simulink model "eml_asteroids"  (R2015a)
settings: Solver=FixedStepDiscrete  StartTime=0.0  StopTime=inf  FixedStep=1  RelTol=1e-3
StopFcn:
  | obj = findobj( 'Tag', 'asteroids_fig');
  | if ~isempty(obj),
  |    close(obj);
  | end;
libraries: simulink x2
(part 1 of 2)
CloseFcn:
  | rtwprivate ssgencode ModelCloseRequest asteroids_fixpt2
Description:
  | MATLAB fixed point version of the classic Asteroids game.
  | 
  | The classic Asteroids game. Even though it is purely fictitious (and not even physically
  | correct), it is nevertheless a complicated dynamic system including collisions,
  | rotating polygons and gaming logic.
  | 
  | This version is using MATLAB Function block and fixed point to demonstrate that all the
  | computations can be done without use of floating point math. Only the "Plot" block
  | in this model contains doubles for displaying and figure handling.
  | 
  | The orange blocks are the core of the simulation and the yellow block is responsible for
  | displaying the results. The blue blocks are managing the input controls, i.e. the space
  | ship rotation, thrust and firing.
  | 
  | Except for the "Plot" visualization block's use of plotting routines, all of the
  | MATLAB Function blocks in this model support code generation with
  | Real-Time Workshop and Real-Time Workshop Embedded Coder.
  | 
  |   Demo Requirements
  | 
  | During this demonstration, Simulink generates code for the simulation in a Simulink
  | project directory created in the current working directory (pwd). If you do not want
  | to affect the current directory (or if you cannot) generate files in this directory, you
  | should change your working directory.
settings Model: CovSFcnEnable=off  ExtModeAutoUpdateStatusClock=off  Creator=The MathWorks, Inc.  LastModifiedBy=ktrinh
settings DataIOCC: SaveFormat=Structure
settings OptimizationCC: ExpressionDepthLimit=2147483647  InitFltsAndDblsToZero=on  EfficientMapNaN2IntZero=off  BufferReusableBoundary=off
settings DebuggingCC: SaveWithParameterizedLinksMsg=none  UnderspecifiedInitializationDetection=Classic  MergeDetectMultiDrivingBlocksExec=none  CheckExecutionContextPreStartOutputMsg=on  CheckExecutionContextRuntimeOutputMsg=on  SignalResolutionControl=TryResolveAllWithWarning  SolverPrmCheckMsg=warning  MultiTaskDSMMsg=warning  MultiTaskCondExecSysMsg=none  SigSpecEnsureSampleTimeMsg=none  IntegerOverflowMsg=none  FcnCallInpInsideContextMsg=EnableAllAsWarning  BusObjectLabelMismatch=none  StateNameClashWarn=warning  IntegerSaturationMsg=none
settings SFSimCC: SimParseCustomCode=off
settings GRTTargetCC: TargetFcnLib=ansi_tfl_tmw.mat  CombineOutputUpdateFcns=off  GRTInterface=on

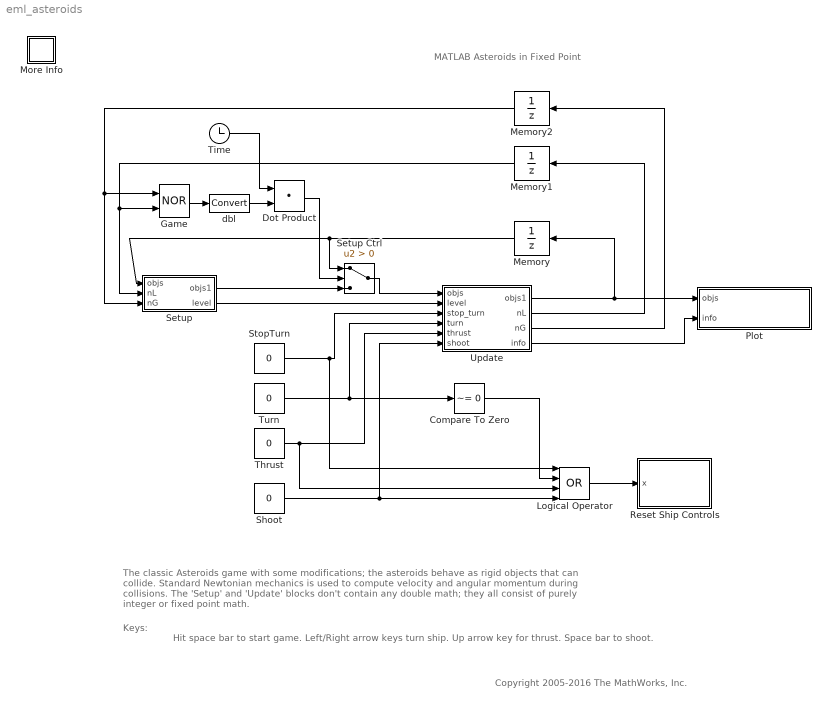
== system eml_asteroids ==
  note: MATLAB Asteroids in Fixed Point
  note: The classic Asteroids game with some modifications; the asteroids behave as rigid objects that can collide.
      | Standard Newtonian mechanics is used to compute velocity and angular momentum during collisions. The 'Setup'
      | and 'Update' blocks don't contain any double math; they all consist of purely integer or fixed point math.
  note: Hit space bar to start game. Left/Right arrow keys turn ship. Up arrow key for thrust.
      | Space bar to shoot.
  note: Keys:
  note: Copyright 2005-2016 The MathWorks, Inc.
  Compare To Zero : simulink/Logic and Bit Operations/Compare To Zero  relop=~=  OutDataTypeStr=boolean  ZeroCross=off
  Dot Product : DotProduct  InputSameDT=on  OutDataTypeStr=Inherit: Inherit via internal rule
  Game : Logic  Operator=NOR  AllPortsSameDT=off  OutDataTypeStr=boolean
  Logical Operator : Logic  Operator=OR  Inputs=4  AllPortsSameDT=off  OutDataTypeStr=boolean
  Memory : UnitDelay  SampleTime=-1
  Memory1 : UnitDelay  SampleTime=-1
  Memory2 : UnitDelay  SampleTime=-1
  More Info : Subsystem
      mask Display: disp('?')
  Plot : MATLAB Function  TreatAsAtomicUnit=on
      settings: PermitHierarchicalResolution=ParametersOnly
  Reset Ship Controls : MATLAB Function  TreatAsAtomicUnit=on
      settings: PermitHierarchicalResolution=ParametersOnly
  Setup : Subsystem
  Setup Ctrl : Switch  Criteria=u2 > Threshold  ZeroCross=off
  Shoot : Constant  Value=0  OutDataTypeStr=boolean
  StopTurn : Constant  Value=0  OutDataTypeStr=boolean
  Thrust : Constant  Value=0  OutDataTypeStr=boolean
  Time : Clock
  Turn : Constant  Value=0  OutDataTypeStr=int32
  Update : Subsystem
  dbl : DataTypeConversion
  wires:
  Time/1 -> Dot Product/1
  Memory/1 -> Setup Ctrl/1, Setup/1(objs)
  Setup Ctrl/1 -> Update/1(objs)
  Turn/1 -> Compare To Zero/1, Update/4(turn)
  Thrust/1 -> Logical Operator/3, Update/5(thrust)
  Logical Operator/1 -> Reset Ship Controls/1(x)
  StopTurn/1 -> Logical Operator/1, Update/3(stop_turn)
  Shoot/1 -> Logical Operator/4, Update/6(shoot)
  Update/1(objs1) -> Plot/1(objs), Memory/1
  Update/2(nL) -> Memory1/1
  Memory1/1 -> Game/2, Setup/2(nL)
  Dot Product/1 -> Setup Ctrl/2
  dbl/1 -> Dot Product/2
  Game/1 -> dbl/1
  Compare To Zero/1 -> Logical Operator/2
  Setup/1(objs1) -> Setup Ctrl/3
  Memory2/1 -> Game/1, Setup/3(nG)
  Update/3(nG) -> Memory2/1
  Update/4(info) -> Plot/2(info)
  Setup/2(level) -> Update/2(level)

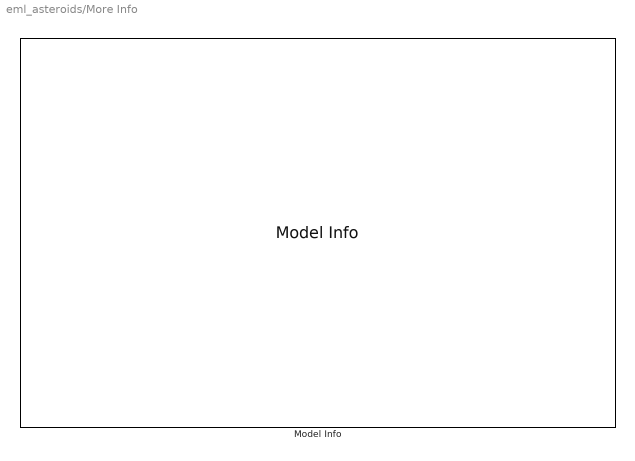
== system eml_asteroids/More Info ==
  Model Info : simulink/Model-Wide Utilities/Model Info  Frame=on  DisplayStringWithTags=|  HorizontalTextAlignment=Left  LeftAlignmentValue=0.02
      | Model Description:
      | -------------------
      | 
      | %<Description>

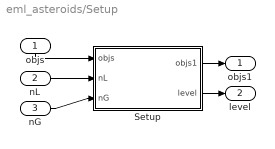
== system eml_asteroids/Setup ==
  objs : Inport
  nL : Inport  Port=2
  nG : Inport  Port=3
  Setup : MATLAB Function  TreatAsAtomicUnit=on
      settings: PermitHierarchicalResolution=ParametersOnly
  objs1 : Outport
  level : Outport  Port=2
  wires:
  objs/1 -> Setup/1(objs)
  nL/1 -> Setup/2(nL)
  nG/1 -> Setup/3(nG)
  Setup/1(objs1) -> objs1/1
  Setup/2(level) -> level/1

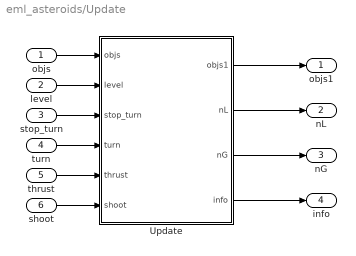
== system eml_asteroids/Update ==
  objs : Inport
  level : Inport  Port=2
  stop_turn : Inport  Port=3
  turn : Inport  Port=4
  thrust : Inport  Port=5
  shoot : Inport  Port=6
  Update : MATLAB Function  TreatAsAtomicUnit=on
      settings: PermitHierarchicalResolution=ParametersOnly
  objs1 : Outport
  nL : Outport  Port=2
  nG : Outport  Port=3
  info : Outport  Port=4
  wires:
  stop_turn/1 -> Update/3(stop_turn)
  turn/1 -> Update/4(turn)
  thrust/1 -> Update/5(thrust)
  shoot/1 -> Update/6(shoot)
  objs/1 -> Update/1(objs)
  Update/1(objs1) -> objs1/1
  level/1 -> Update/2(level)
  Update/2(nL) -> nL/1
  Update/3(nG) -> nG/1
  Update/4(info) -> info/1

== matlab function eml_asteroids/Setup/Setup ==
  data: objs input fixdt('sfix32_En12'); nL input boolean; objs1 output fixdt('sfix32_En12'); nG input boolean; level output fixdt('sfix32_En12')
function [objs1,level] = setup(objs,nL,nG)

% nL = nextLevel

my_fimath = fimath('MaxProductWordLength',32,'MaxSumWordLength',32,...
                   'ProductFractionLength',12,'ProductMode','SpecifyPrecision',...
                   'SumFractionLength',12,'SumMode','SpecifyPrecision');
my_fitype = numerictype(1,32,12);

persistent level0;
persistent objs0;

maxobjs = 64;

initial = false;

if isempty(level0)
    level0 = fi(0,my_fitype,my_fimath);
    nL = true;
    initial = true;
end

if nG
    level0 = fi(0,my_fitype,my_fimath);
    nL = true;
end

if nL
    level0 = level0 + 1;
end

level = level0;

objs0 = fi(objs,my_fitype,my_fimath);

if isempty(objs0)
    objs0 = fi(zeros(11,maxobjs),my_fitype,my_fimath);
end

if nG
    % Delete all objects that is not a ship
    for i = 1:maxobjs
        if objs0(1,i) ~= 2 % ship id
            objs0(1,i) = 0;
        end
    end
end

if nL
    if level0 < 5
        level0_int = fi(level0,numerictype(1,16,0));
        n = int32(level0_int) + 1;
    else
        n = int32(5);
    end
 
    if initial
        n = int32(20);
    end
 
    for z = int32(1):n
        objs0 = add_asteroid(objs0,initial);
    end
       
    % Move objects so two objects never collide
    
     for z = int32(1):n
         x = objs0(2,z);
         y = objs0(3,z);
         r = objs0(10,z);
         q = true;
         while q
             c = false;
             for k = int32(1):n
                 if z ~= k
                     xk = objs0(2,k);
                     yk = objs0(3,k);
                     rk = objs0(10,k);
                     dx = x-xk;
                     ddx = x*xk;
                     dy = y-yk;
                     rrk = r+rk;
                     if dx*dx+dy*dy < rrk*rrk
                         c = true;
                         break;
                     end
                 end
             end
             q = c;
             if q
                 x = fi(400 * fi_rand(),my_fitype,my_fimath);
                 y = fi(400 * fi_rand(),my_fitype,my_fimath);
                 objs0(2,z) = x;
                 objs0(3,z) = y;
             end
         end
     end  
end
objs1 = objs0;

function [objs1,index] = add_object(objs,id,r)
    my_fimath = fimath('MaxProductWordLength',32,'MaxSumWordLength',32);
    my_fitype = numerictype(1,32,20);

    x = 400 * fi_rand();
    y = 400 * fi_rand();
    arg = fi_rand()*2*pi;
    vx = fi_rand()*6 - 3;
    vy = fi_rand()*6 - 3;
    varg = fi_rand()*0.2 - 0.1;
    collidable = 1;
    i = add_new(objs);
    col = double('w');
    cnt = 0;
    objs(:,i) = fi([id x y arg vx vy varg collidable col r cnt]',my_fitype,my_fimath);
    objs1 = objs;
    index = i;

function objs1 = add_asteroid(objs,initial)
    r = fi_rand() * 15 + 8;
    if ~initial
        r(:) = 30;
    end 
    [objs1,i] = add_object(objs,int32(1),r);
    objs1(5,i) = objs1(5,i)*0.1;
    objs1(6,i) = objs1(6,i)*0.1;
    objs1(7,i) = objs1(7,i)*0.1;

function r = fi_rand()

persistent state;

my_fimath0 = fimath('MaxProductWordLength',32,'MaxSumWordLength',32,...
                    'ProductFractionLength',32,'ProductMode','SpecifyPrecision',...
                    'SumFractionLength',32,'SumMode','SpecifyPrecision',...
                    'OverflowMode','wrap');
my_fitype0 = numerictype(0,32,32);
                
my_fimath = fimath('MaxProductWordLength',32,'MaxSumWordLength',32,...
                   'ProductFractionLength',12,'ProductMode','SpecifyPrecision',...
                   'SumFractionLength',12,'SumMode','SpecifyPrecision');

my_fitype = numerictype(1,32,12);

if isempty(state)
    state = fi(0,my_fitype0,my_fimath0);
end

state = state * 34567.27491803 + 43178.421727917;

r = fi(state,my_fitype,my_fimath);

function index = add_new(objs)
    maxobjs = 64;
    index = int32(-1);
    for i = 1:maxobjs,
        if objs(1,i) == 0,
            index = int32(i);
            return
        end
    end

== matlab function eml_asteroids/Update/Update ==
  settings: updateMethod=DISCRETE
  data: objs input fixdt('sfix32_En12') size=[11,64]; level input fixdt('sfix32_En12'); stop_turn input boolean; turn input int32 size=1; objs1 output fixdt('sfix32_En12') size=[11,64]; nL output boolean; nG output boolean; info output fixdt('sfix32_En12'); thrust input boolean; shoot input boolean
function [objs1,nL,nG,info] = update(objs, level, stop_turn, turn, thrust, shoot)

persistent stop;
persistent thrust_cnt;
persistent turn_cnt;
persistent turn_dir;
persistent ship_cnt;
persistent ship_destroyed_cnt;
persistent level_complete_cnt;
persistent score;

my_fimath = fimath('MaxProductWordLength',32,'MaxSumWordLength',32,...
                   'ProductFractionLength',12,'ProductMode','SpecifyPrecision',...
                   'SumFractionLength',12,'SumMode','SpecifyPrecision');
my_fitype = numerictype(1,32,12);

objs1 = fi(objs,my_fitype,my_fimath);
nL = false;
nG = false;

if isempty(score)
    score = fi(0,my_fitype,my_fimath);
end

%
% stop is used for debugging. It is convenient to "freeze" the
% updates.
%
if isempty(stop)
    stop = false;
end

if isempty(ship_cnt)
    ship_cnt = fi(0,my_fitype,my_fimath);
end

if isempty(thrust_cnt)
    thrust_cnt = fi(0,my_fitype,my_fimath);
end

if isempty(turn_cnt) || stop_turn
    turn_cnt = fi(0,my_fitype,my_fimath);
    turn_dir = int32(0);
end

if isempty(ship_destroyed_cnt)
    ship_destroyed_cnt = fi(0,my_fitype,my_fimath);
end

if isempty(level_complete_cnt)
    level_complete_cnt = fi(0,my_fitype,my_fimath);
end

if level_complete_cnt > 200
    level_complete_cnt = fi(0,my_fitype,my_fimath);
    nL = true;
end

if turn ~= 0
    turn_cnt = fi(3,my_fitype,my_fimath);
    turn_dir = turn;
end

info = [level ship_cnt score];

if stop
    return
end

min_x = fi(0,my_fitype,my_fimath) - 20;
max_x = fi(400,my_fitype,my_fimath) + 20;
min_y = fi(0,my_fitype,my_fimath) - 20;
max_y = fi(400,my_fitype,my_fimath) + 20;
width = max_x - min_x;
height = max_y - min_y;

origin_x = (max_x + min_x) * 0.5;
origin_y = (max_y + min_y) * 0.5;

if ship_destroyed_cnt > 0
    ship_destroyed_cnt = ship_destroyed_cnt - 1;
end

% Make sure thrust is at the same position as ship
maxobjs = int32(64);

ship_index = int32(0);
thrust_index = int32(0);
no_asteroids = true;
for i = int32(1):maxobjs
    if objs1(1,i) == 2 % space ship id
        ship_index = int32(i);
    end
    if objs1(1,i) == 5 % thrust id
        thrust_index = int32(i);
    end
    if objs1(1,i) == 1 % asteroid id
        no_asteroids = false;
    end
end

ship_exists = ship_index > 0;

if ship_destroyed_cnt <= 0 && ship_cnt > 0 && ~ship_exists
    if is_space_empty(objs1,origin_x,origin_y,40)
        [objs1,ship_index] = add_ship(objs1,origin_x,origin_y);
        ship_cnt = ship_cnt - 1;
        ship_exists = true;
    end
end

if ~ship_exists && shoot && ship_cnt == 0
    ship_cnt = fi(3,my_fitype,my_fimath);
    score = fi(0,my_fitype,my_fimath);
    nG = true;
end

if thrust ~= 0 && thrust_cnt == 0 && ship_index > 0
    thrust_cnt = fi(7,my_fitype,my_fimath);
    [objs1,thrust_index] = add_thrust(objs1);
end

if no_asteroids && ship_index > 0
    level_complete_cnt = level_complete_cnt + 1;
end
    
if thrust_index > 0 && ship_index > 0
    objs1(2:7,thrust_index) = objs1(2:7,ship_index);
end

% fprintf(1,'i=%d id=%d r=%d\n', i, double(objs1(1,i)), double(objs1(2,i)));

%
% Start updating all objects
%

for i = int32(1):maxobjs
    id = objs1(1,i);
%    fprintf(1,'i=%d id=%d r=%d\n', i, double(id), double(objs1(1,i)));
    if id == 0 % marked deleted
        continue
    end
    x = objs1(2,i);
    y = objs1(3,i);
    arg = objs1(4,i);
    vx = objs1(5,i);
    vy = objs1(6,i);
    varg = objs1(7,i);
    collidable = objs1(8,i);
    color = objs1(9,i);
    r = objs1(10,i);
    cnt = objs1(11,i);
        
    if cnt > 0
        cnt = cnt - 1;
        objs1(11,i) = cnt;
        if cnt <= 0 % delete object
            objs1(1,i) = 0;
            continue
        end
    end
    
    if id == 2 % space ship
        
        if turn_cnt > 0
            turn_cnt = turn_cnt - 1;
            if turn_dir == -1
                varg = fi(-0.1,numerictype(varg),fimath(varg));
            elseif turn_dir == 1
                varg = fi(0.1,numerictype(varg),fimath(varg));
            else
                varg = fi(0,numerictype(varg),fimath(varg));
            end
        else
            varg = fi(0,numerictype(varg),fimath(varg));
        end
        objs1(7,i) = varg;
        
        if thrust_cnt > 0
            thrust_cnt = thrust_cnt - 1;            
            if thrust_cnt == 6
                vx = vx + cos(arg)*0.3;
                vy = vy + sin(arg)*0.3;
            end
            objs1(5,i) = vx;
            objs1(6,i) = vy;
        end
        
        if shoot ~= 0 && ship_exists
            missile_cnt = fi(0,my_fitype,my_fimath);
            for j = int32(1):maxobjs
                if objs(1,j) == 3
                    missile_cnt = missile_cnt + 1;
                end
            end
            if missile_cnt < 3
                mx = x + (r+2)*cos(arg);
                my = y + (r+2)*sin(arg);
                mvx = vx + 3*cos(arg);
                mvy = vy + 3*sin(arg);
                objs1 = add_missile(objs1,mx,my,mvx,mvy,arg);
                missile_cnt = missile_cnt + 1;
            end
        end
    end
    
    arg = arg + varg;
    x = x + vx;
    y = y + vy;    
    
    while arg >= 2*pi, arg = arg - 2*pi; end
    while arg < 0, arg = arg + 2*pi; end

    objs1(2,i) = x;
    objs1(3,i) = y;
    objs1(4,i) = arg;
    
    while x > max_x
        x = x - width;
        objs1(2,i) = x;
        objs1 = move_to_empty_space(objs1,i,int32(0),int32(10),min_x,max_x,min_y,max_y);
    end
    while x < min_x
        x = x + width;
        objs1(2,i) = x;
        objs1 = move_to_empty_space(objs1,i,int32(0),int32(10),min_x,max_x,min_y,max_y);
    end
    while y > max_y
        y = y - height; 
        objs1(3,i) = y;
        objs1 = move_to_empty_space(objs1,i,int32(10),int32(0),min_x,max_x,min_y,max_y);
    end
    while y < min_y
        y = y + height; 
        objs1(3,i) = y;
        objs1 = move_to_empty_space(objs1,i,int32(10),int32(0),min_x,max_x,min_y,max_y);
    end
    
    [xs ys n] = get_object_data(objs1(:,i));
    
    for j = int32(1):maxobjs
        if objs1(1,j) == 0 % object marked deleted
            continue
        end
        collidable_j = objs1(8,j);
        if i ~= j && collidable ~= 0 && collidable_j ~= 0 && collides(objs1(:,i),objs1(:,j))

            if (objs1(1,i) == 3 && objs1(1,j) == 1) || ...
               (objs1(1,i) == 1 && objs1(1,j) == 3) % if missile + asteroid
                [dir_x,dir_y] = get_any_dir;
                if objs1(1,i) == 3
                    x0 = objs1(2,i); y0 = objs1(3,i);
                    objs1(:,i) = objs1(:,j);
                else
                    x0 = objs1(2,j); y0 = objs1(3,j);
                    objs1(:,j) = objs1(:,i);
                end
                vel = fi(2,my_fitype,my_fimath);
                vel = vel*fi_rand() + 1;
                asteroid_size = objs1(10,i);
                objs1(10,i) = objs1(10,i) * 0.5;
                objs1(10,j) = objs1(10,i);
                if objs1(10,i) < 4
                    objs1(1,i) = 0;
                    objs1(1,j) = 0;
                else
                    objs1(4,i) = objs1(4,i) + vel*dir_x;
                    objs1(5,i) = objs1(5,i) + vel*dir_y;
                    objs1(4,j) = objs1(4,j) - vel*dir_x;
                    objs1(5,j) = objs1(5,j) - vel*dir_y;
                    objs1(2,i) = objs1(2,i) + objs1(10,i)*dir_x;
                    objs1(3,i) = objs1(3,i) + objs1(10,i)*dir_y;
                    objs1(2,j) = objs1(2,j) - objs1(10,i)*dir_x;
                    objs1(3,j) = objs1(3,j) - objs1(10,i)*dir_y;
                end
                objs1 = add_explosion(objs1,x0,y0,int32(40));

                if asteroid_size >= 25
                    score = score + 20;
                elseif asteroid_size >= 13
                    score = score + 50;
                else
                    score = score + 100;
                end

                continue
            end

            ship_index = int32(-1);
            ship_vx = fi(0,my_fitype,my_fimath);
            ship_vy = fi(0,my_fitype,my_fimath);
            ship_varg = fi(0,my_fitype,my_fimath);
            if (objs1(1,i) == 2 || objs1(1,j) == 2) % if ship + something else
                if objs1(1,i) == 2
                    ship_index = int32(i);
                else
                    ship_index = int32(j);
                end
                ship_vx = objs1(5,ship_index);
                ship_vy = objs1(6,ship_index);
                ship_varg = objs1(7,ship_index);
            end

%            objs1(9,i) = double('r');
            [objs1(:,i),objs1(:,j)] = do_collision(objs1(:,i),objs1(:,j));

            if ship_index ~= -1
                ship_vx = ship_vx - objs1(5,ship_index);
                ship_vy = ship_vy - objs1(6,ship_index);
                ship_varg = ship_varg - objs1(7,ship_index);
                ship_vr = ship_varg*ship_r();
                % If ship gained to much energy in the collison we'll destroy it
                delta = sqrt(ship_vx*ship_vx+ship_vy*ship_vy+ship_varg*ship_varg);
                if delta >= 0.2 % Empirically tested (it feels right)
                    objs1(1,ship_index) = 0; % remove ship
                    ship_destroyed_cnt = fi(100,my_fitype,my_fimath);
                    objs1 = add_explosion(objs1,objs1(2,ship_index),objs1(3,ship_index),int32(100));
                end
            end
            
%            stop = true;
            break
        else
%            objs1(9,i) = double('w');
        end
    end
end

function b = is_space_empty(objs,x,y,r)
    maxobjs = 64;
    for j = 1:maxobjs
        if objs(8,j) ~= 0 && objs(1,j) ~= 0 ...
            radius = objs(10,j);
            dx = objs(2,j) - x;
            dy = objs(3,j) - y;
            if dx*dx+dy*dy < (r+radius)*(r+radius)
                b = false;
                return
            end
        end
    end
    b = true;

function objs1 = move_to_empty_space(objs,obj_i,dx,dy,min_x,max_x,min_y,max_y)
    maxobjs = 64;
    width = max_x - min_x;
    height = max_y - min_y;
    objs1 = objs;
    some_collision = true;
    wraps = int32(0);
    if objs1(8,obj_i) == 0
        return
    end
    while some_collision && wraps < 2
        some_collision = false;
        for j = 1:maxobjs
            if objs1(1,j) == 0
                continue
            end
            if obj_i ~= j && objs1(8,j) ~= 0 && collides(objs1(:,obj_i),objs1(:,j))
                x = objs1(2,obj_i);
                y = objs1(3,obj_i);
                x = x + dx;
                y = y + dy;
                while x > max_x, x = x - width; wraps = wraps + 1; end
                while x < min_x, x = x + width; wraps = wraps + 1; end
                while y > max_y, y = y - height; wraps = wraps + 1; end
                while y < min_y, y = y + height; wraps = wraps + 1; end
                objs1(2,obj_i) = x;
                objs1(3,obj_i) = y;
                some_collision = true;
            end
        end
    end

function r = fi_rand()

persistent state;

my_fimath0 = fimath('MaxProductWordLength',32,'MaxSumWordLength',32,...
                    'ProductFractionLength',32,'ProductMode','SpecifyPrecision',...
                    'SumFractionLength',32,'SumMode','SpecifyPrecision',...
                    'OverflowMode','wrap');
my_fitype0 = numerictype(0,32,32);
                
my_fimath = fimath('MaxProductWordLength',32,'MaxSumWordLength',32,...
                   'ProductFractionLength',12,'ProductMode','SpecifyPrecision',...
                   'SumFractionLength',12,'SumMode','SpecifyPrecision');

my_fitype = numerictype(1,32,12);

if isempty(state)
    state = fi(0,my_fitype0,my_fimath0);
end

state = state * 34567.27491803 + 43178.421727917;

r = fi(state,my_fitype,my_fimath);

%
% get any direction
%


function [dx,dy] = get_any_dir
    arg = fi_rand()*2*pi;
    dx = cos(arg);
    dy = sin(arg);

%
% do_collision
%
% Compute new momentum for objects
%

function [obj1,obj2] = do_collision(obj1,obj2)

[px,py] = collision_point(obj1,obj2);
[nx,ny] = collision_normal(obj1,obj2);
n = [nx ny];
p = [px py];

c = true;

cnt = int32(0);

while c
    [obj1,obj2] = do_collision0(obj1,obj2,p,n);

    c = collides(obj1,obj2);
    if c
        q = fi_rand();
        arg = fi(q,numerictype(p),fimath(p)) * 2 * pi;
        n = n * [cos(arg) sin(arg); -sin(arg) cos(arg)];
        cnt = cnt + 1;
        if cnt > 10
%            disp('failed!');
            break;
        end
    end
end

function [obj1,obj2] = do_collision0(obj1,obj2,p,n)

px = p(1);
py = p(2);
nx = n(1);
ny = n(2);

i1 = get_inertia(obj1);
m1 = get_mass(obj1);
x1 = obj1(2);
y1 = obj1(3);
vx1 = obj1(5);
vy1 = obj1(6);
w1 = obj1(7);
r1 = obj1(10);

i2 = get_inertia(obj2);
m2 = get_mass(obj2);
x2 = obj2(2);
y2 = obj2(3);
vx2 = obj2(5);
vy2 = obj2(6);
w2 = obj2(7);
r2 = obj2(10);

%
% Before we do anything, let's undo the collision point so
% objects don't get stuck because we compute the collision
% normal slightly wrong.
%

obj1(2) = obj1(2) - vx1;
obj1(3) = obj1(3) - vy1;
obj1(4) = obj1(4) - w1;
obj2(2) = obj2(2) - vx2;
obj2(3) = obj2(3) - vy2;
obj2(4) = obj2(4) - w2;


v1 = [vx1 vy1];
v2 = [vx2 vy2];
r1p = [px-x1 py-y1];
r2p = [px-x2 py-y2];

w1r1p = cross([0 0 w1],[r1p 0]);
w2r2p = cross([0 0 w2],[r2p 0]);

v1p = v1 + w1r1p(1:2);
v2p = v2 + w2r2p(1:2);

v21 = v1p - v2p;

e = 1.00;

xx1 = cross([r1p 0],[n 0]);
xx2 = cross([r2p 0],[n 0]);

j1 = (-(1+e)*v21) * n';
j2 = divide(numerictype(m1),1,m1) + ...
     divide(numerictype(m2),1,m2) + ...
     divide(numerictype(xx1),(xx1 * xx1'),i1) + ...
     divide(numerictype(xx2),(xx2 * xx2'),i2);

j = divide(numerictype(j1),j1,j2);

new_v1 = v1 + j * divide(numerictype(n),n,m1);
new_v2 = v2 - j * divide(numerictype(n),n,m2);

new_w1 = w1 + divide(numerictype(j),j,i1)*xx1(3);
new_w2 = w2 - divide(numerictype(j),j,i2)*xx2(3);

obj1(5) = new_v1(1);
obj1(6) = new_v1(2);
obj1(7) = new_w1;

obj2(5) = new_v2(1);
obj2(6) = new_v2(2);
obj2(7) = new_w2;

obj1(2) = obj1(2) + new_v1(1);
obj1(3) = obj1(3) + new_v1(2);
obj1(4) = obj1(4) + new_w1;

obj2(2) = obj2(2) + new_v2(1);
obj2(3) = obj2(3) + new_v2(2);
obj2(4) = obj2(4) + new_w2;
   
%
% add object
%

function [objs1,index] = add_object(objs,id,r,x,y,vx,vy,arg,col)
    my_fimath = fimath('MaxProductWordLength',32,'MaxSumWordLength',32,...
                       'ProductFractionLength',12,'ProductMode','SpecifyPrecision',...
                       'SumFractionLength',12,'SumMode','SpecifyPrecision');
    my_fitype = numerictype(1,32,12);
    varg = 0;
    collidable = 1;
    index = add_new(objs);
    if nargin < 9
        ficol = fi(int32('w'),my_fitype,my_fimath);
    else
        ficol = fi(int32(col),my_fitype,my_fimath);
    end
    objs(:,index) = fi([id x y arg vx vy varg collidable ficol r -1]',my_fitype,my_fimath);
    objs1 = objs;

function [objs1,index] = add_ship(objs,x,y)
    my_fimath = fimath('MaxProductWordLength',32,'MaxSumWordLength',32,...
                       'ProductFractionLength',12,'ProductMode','SpecifyPrecision',...
                       'SumFractionLength',12,'SumMode','SpecifyPrecision');
    my_fitype = numerictype(1,32,12);
    [objs1,index] = add_object(objs,2,15,x,y,0,0,fi(pi/2,my_fitype,my_fimath),'g');

function [objs1,index] = add_thrust(objs)
    [objs1,index] = add_object(objs,5,15,0,0,0,0,0,'y');
    objs1(11,index) = 15; % Life time
    objs1(8,index) = 0; % not collidable
    
function objs1 = add_missile(objs,x,y,vx,vy,arg)
    [objs1,index] = add_object(objs,3,4,x,y,vx,vy,arg,'y');
    objs1(11,index) = 50; % Life time

function obj = new_explosion(x,y,n)
    my_fimath = fimath('MaxProductWordLength',32,'MaxSumWordLength',32,...
                       'ProductFractionLength',12,'ProductMode','SpecifyPrecision',...
                       'SumFractionLength',12,'SumMode','SpecifyPrecision');
    my_fitype = numerictype(1,32,12);
    obj = fi([4 x y 0 0 0 0 0 double('w') n 2]',my_fitype,my_fimath);
    
function objs1 = add_explosion(objs,x,y,n)
    index = add_new(objs);
    obj = new_explosion(x,y,n);
    objs1 = objs;
    objs1(:,index) = obj;
    
function index = add_new(objs)
    my_fimath = fimath('MaxProductWordLength',32,'MaxSumWordLength',32,...
                       'ProductFractionLength',12,'ProductMode','SpecifyPrecision',...
                       'SumFractionLength',12,'SumMode','SpecifyPrecision');
    my_fitype = numerictype(1,32,12);
    maxobjs = 64;
    index = int32(-1);
    for i = 1:maxobjs,
        if objs(1,i) == 0
            index = int32(i);
            return
        end
    end
    feval('error','overflow objects');

function n = get_number(objs)    
    n = add_new(objs);

%
% get_object_data
%
% Get point data given object
%
function [xs ys n] = get_object_data(obj)

id = obj(1);
x = obj(2);
y = obj(3);
arg = obj(4);
r = obj(10);

xs = fi([0 0 0 0 0 0 0 0 0 0 0 0 0 0 0 0],numerictype(x),fimath(x));
ys = fi([0 0 0 0 0 0 0 0 0 0 0 0 0 0 0 0],numerictype(y),fimath(y));
n = int32(0);
if id == 1,
    asteroid_x0 = asteroid_x();
    asteroid_y0 = asteroid_y();
    asteroid_r0 = asteroid_r();
    f = divide(numerictype(r),r,asteroid_r0);
    n = int32(size(asteroid_x0,1));
    xs(1:n) = x + f * asteroid_x0 * cos(arg) - f * asteroid_y0 * sin(arg);
    ys(1:n) = y + f * asteroid_x0 * sin(arg) + f * asteroid_y0 * cos(arg);
elseif id == 2
    ship_x0 = ship_x();
    ship_y0 = ship_y();
    ship_r0 = ship_r();
    f = divide(numerictype(r),r,ship_r0);
    n = int32(size(ship_x0,1));
    xs(1:n) = x + f * ship_x0 * cos(arg) - f * ship_y0 * sin(arg);
    ys(1:n) = y + f * ship_x0 * sin(arg) + f * ship_y0 * cos(arg);    
else % id == 3
    missile_x0 = missile_x();
    missile_y0 = missile_y();
    missile_r0 = missile_r();
    f = divide(numerictype(r),r,missile_r0);
    n = int32(size(missile_x0,1));
    xs(1:n) = x + f * missile_x0 * cos(arg) - f * missile_y0 * sin(arg);
    ys(1:n) = y + f * missile_x0 * sin(arg) + f * missile_y0 * cos(arg);    
end

%
% asteroid_x
% asteroid_y
%
% Returning asteroid x and y data
%

function r = asteroid_x
    my_fimath = fimath('MaxProductWordLength',32,'MaxSumWordLength',32,...
                       'ProductFractionLength',12,'ProductMode','SpecifyPrecision',...
                       'SumFractionLength',12,'SumMode','SpecifyPrecision');
    my_fitype = numerictype(1,32,12);
    r = fi([2 10 20 17 7 16 12 -7 -17 -21 -14 -8 -7]',my_fitype,my_fimath);

function r = asteroid_y
    my_fimath = fimath('MaxProductWordLength',32,'MaxSumWordLength',32,...
                       'ProductFractionLength',12,'ProductMode','SpecifyPrecision',...
                       'SumFractionLength',12,'SumMode','SpecifyPrecision');
    my_fitype = numerictype(1,32,12);
    r = fi([18 22 5 -4 -6 -10 -17 -19 -13 3 17 11 23]',my_fitype,my_fimath);

function r = asteroid_r
    my_fimath = fimath('MaxProductWordLength',32,'MaxSumWordLength',32,...
                       'ProductFractionLength',12,'ProductMode','SpecifyPrecision',...
                       'SumFractionLength',12,'SumMode','SpecifyPrecision');
    my_fitype = numerictype(1,32,12);
    r = fi(22,my_fitype,my_fimath);

function r = ship_x
    my_fimath = fimath('MaxProductWordLength',32,'MaxSumWordLength',32,...
                       'ProductFractionLength',12,'ProductMode','SpecifyPrecision',...
                       'SumFractionLength',12,'SumMode','SpecifyPrecision');
    my_fitype = numerictype(1,32,12);
    r = fi([-4,-2,-2,-4,8]',my_fitype,my_fimath);
    
function r = ship_y
    my_fimath = fimath('MaxProductWordLength',32,'MaxSumWordLength',32,...
                       'ProductFractionLength',12,'ProductMode','SpecifyPrecision',...
                       'SumFractionLength',12,'SumMode','SpecifyPrecision');
    my_fitype = numerictype(1,32,12);
    r = fi([4,1,-1,-4,0]',my_fitype,my_fimath);

function r = ship_r
    my_fimath = fimath('MaxProductWordLength',32,'MaxSumWordLength',32,...
                       'ProductFractionLength',12,'ProductMode','SpecifyPrecision',...
                       'SumFractionLength',12,'SumMode','SpecifyPrecision');
    my_fitype = numerictype(1,32,12);
    r = fi(10,my_fitype,my_fimath);
    
function r = missile_x
    my_fimath = fimath('MaxProductWordLength',32,'MaxSumWordLength',32,...
                       'ProductFractionLength',12,'ProductMode','SpecifyPrecision',...
                       'SumFractionLength',12,'SumMode','SpecifyPrecision');
    my_fitype = numerictype(1,32,12);
    r = fi([-4,4]',my_fitype,my_fimath);
    
function r = missile_y
    my_fimath = fimath('MaxProductWordLength',32,'MaxSumWordLength',32,...
                       'ProductFractionLength',12,'ProductMode','SpecifyPrecision',...
                       'SumFractionLength',12,'SumMode','SpecifyPrecision');
    my_fitype = numerictype(1,32,12);
    r = fi([0,0]',my_fitype,my_fimath);

function r = missile_r
    my_fimath = fimath('MaxProductWordLength',32,'MaxSumWordLength',32,...
                       'ProductFractionLength',12,'ProductMode','SpecifyPrecision',...
                       'SumFractionLength',12,'SumMode','SpecifyPrecision');
    my_fitype = numerictype(1,32,12);
    r = fi(8,my_fitype,my_fimath);        

%
% collides(obj1,obj2)
%
% Return true if obj1 collides with obj2.
%
function r = collides(obj1,obj2)
    id1 = obj1(1);
    x1 = obj1(2);
    y1 = obj1(3);
    r1 = obj1(10);
    id2 = obj2(1);
    x2 = obj2(2);
    y2 = obj2(3);
    r2 = obj2(10);
    dx = x2 - x1;
    dy = y2 - y1;
    if (dx*dx + dy*dy) < ((r1+r2)*(r1+r2))
        [xs1 ys1 n1] = get_object_data(obj1);
        [xs2 ys2 n2] = get_object_data(obj2);
        r = polygons_collide(xs1,ys1,n1,xs2,ys2,n2);
    else
        r = false;
    end

%
% I = get_inertia(obj)
%

function I = get_inertia(obj)
    r = obj(10);
    m = get_mass(obj);
    I = divide(numerictype(m),m*r*r,2);
%    I = m;

%
% m = get_mass(obj)
%

function m = get_mass(obj)
    m = obj(10);
    
%
% collision_normal(obj1,obj2)
%

function [nx,ny] = collision_normal(obj1,obj2)
    [xs1 ys1 n1] = get_object_data(obj1);
    [xs2 ys2 n2] = get_object_data(obj2);
    [p,i] = polygons_collide_point(xs1,ys1,n1,xs2,ys2,n2);
    if p == 1
        prev_i = i-1;
        if prev_i == 0
            prev_i = n1;
        end
        dx = xs1(i) - xs1(prev_i);
        dy = ys1(i) - ys1(prev_i);
        l = sqrt(dx*dx+dy*dy);
        nx = divide(numerictype(dy),dy,l);
        ny = -divide(numerictype(dx),dx,l);
    elseif p == 2
        prev_i = i-1;
        if prev_i == 0
            prev_i = n2;
        end
        dx = xs2(i) - xs2(prev_i);
        dy = ys2(i) - ys2(prev_i);
        l = sqrt(dx*dx+dy*dy);
        nx = divide(numerictype(dy),dy,l);
        ny = -divide(numerictype(dx),dx,l);
    else
        nx = fi(0,numerictype(xs1),fimath(ys1));
        ny = fi(0,numerictype(xs1),fimath(ys1));
    end
    
%
% collision_point(obj1,obj2)
%

function [x,y] = collision_point(obj1,obj2)
    [xs1 ys1 n1] = get_object_data(obj1);
    [xs2 ys2 n2] = get_object_data(obj2);
    [p,i] = polygons_collide_point(xs1,ys1,n1,xs2,ys2,n2);
    if p == 1
        x = xs1(i);
        y = ys1(i);
    elseif p == 2
        x = xs2(i);
        y = ys2(i);
    else
        x = fi(0,numerictype(xs1),fimath(xs1));
        y = fi(0,numerictype(ys1),fimath(ys1));
    end

%
% polygons_collide(xs1,ys1,xs2,ys2)
%
% Return true if polygon xs1,ys1 collides with xs2,ys2
%
function r = polygons_collide(xs1,ys1,n1,xs2,ys2,n2)

[p,n] = polygons_collide_point(xs1,ys1,n1,xs2,ys2,n2);
r = p ~= 0;

%
% Return [p,n] if polygons collide where
%     where [p,n] represents the collision point such that
%     p = 1 if the point belongs to the first polygon
%     p = 2 if the point belongs to the second polygon
%     n = the index of the point in the polygon that is
%     the collision point.
%     p = 0 if the polygons do not collide

function [p,n] = polygons_collide_point(xs1,ys1,n1,xs2,ys2,n2)
if n2 > 2
    for i = int32(1):int32(n1)
        if inside_polygon(xs1(i),ys1(i),xs2,ys2,n2)
            p = int32(1);
            n = i;
            return;
        end
    end
end

if n1 > 2
    for i = int32(1):int32(n2)
        if inside_polygon(xs2(i),ys2(i),xs1,ys1,n1)
            p = int32(2);
            n = i;
            return;
        end
    end
end
p = int32(0);
n = int32(0);

%
% inside_polygon (Check if point is inside polygon)
%
% Returns true if point (x0,y0) is inside the polygon
% (xs,ys)
%
function r = inside_polygon(x0,y0,xs,ys,max_n)

if nargin <= 4
    max_n = size(xs,1);
end

cnt = int32(0);
n = max_n;
i = int32(1);
while i <= n
    xi = xs(i);
    yi = ys(i);
    j = i + 1;
    if j == n+1
        j = int32(1);
    end
    xj = xs(j);
    yj = ys(j);
    if line_intersect(x0,y0,10000,y0,xi,yi,xj,yj)
        if is_near(yi,y0) || is_near(yj,y0)
            if is_near(yi,y0)
                i_prev = i - 1;
                if i_prev < 1
                    i_prev = n;
                end 
                i_next = i + 1;
            else
                i_prev = i;
                i_next = j + 1;
                if i_next > n
                    i_next = int32(1);
                end
            end
            c = int32(0);
            while c < n && is_near(ys(i_prev),y0)
                i_prev = i_prev - 1;
                if i_prev < 1
                    i_prev = n;
                end
                c = c + 1;
            end
            c = int32(0);
            while c < n && is_near(ys(i_next),y0)
                i_next = i_next + 1;
                if i_next > n
                    i_next = int32(1);
                end
                c = c + 1;
            end
            if sign(ys(i_next) - y0) ~= sign(ys(i_prev) - y0)
                cnt = cnt + 1;
            end
            if i_next < i
                break
            else
                i = i_next - 1;
                if i < 1
                    i = n;
                end
            end
        else
            cnt = cnt + 1;
        end
    end
    i = i + 1;
end
r = rem(cnt,int32(2)) == 1;

function r = is_near(x,y)
    r = abs(x - y) < 0.1;

%
% line_intersect (Line segment intersection check)
%
% Returns true if line (x1,y1)--(x0,y0) intersects
%                      (x2,y2)--(x3,y3)
%
function r = line_intersect(x0,y0,x1,y1,x2,y2,x3,y3)

r = ((ccw(x0,y0,x1,y1,x2,y2) * ccw(x0,y0,x1,y1,x3,y3)) <= 0) && ...
    ((ccw(x2,y2,x3,y3,x0,y0) * ccw(x2,y2,x3,y3,x1,y1)) <= 0);

%
% ccw (Counter clockwise)
%
% Compare vectors (x1,y1) and (x2,y2) w.r.t. (x0,y0) and
% determine whether we visit them clockwise or counter
% clockwise.
%
function r = ccw( x0, y0, x1, y1, x2, y2 )
    dx1 = x1 - x0;
    dy1 = y1 - y0;
    dx2 = x2 - x0;
    dy2 = y2 - y0;
    q = dx1*dy2 - dy1*dx2;
    if q > 0
         r = int32(1);
    elseif q < 0
         r = int32(-1);
    else
        if ((dx1*dx2 < 0) || ((dy1*dy2) < 0))
            r = int32(-1);
        elseif ((dx1*dx1+dy1*dy1) < (dx2*dx2+dy2*dy2))
            r = int32(1);
        else
            r = int32(0);
        end
    end

%
% Currently, sign is not implemented for fi
%

function y = sign(x)
    if x < 0
        y = int32(-1);
    elseif x > 0
        y = int32(1);
    else
        y = int32(0);
    end
    
%
% Currently, sqrt is not implemented for fi
%

function y = sqrt(x)
    % Compute using Newton-Raphson.
    % First compute a good guess
    q = fi(1,numerictype(x),fimath(x));
    g = fi(1,numerictype(x),fimath(x));
    if x > 1
        while q < x
            q = q*4;
            g = g*2;
        end
    else
        while q > x
            q = divide(numerictype(q),q,4);
            g = divide(numerictype(g),g,2);
        end
    end
    y = g;
    for i = 1:4
        y = divide(numerictype(y),(y + divide(numerictype(y),x,y)),2);
    end

%
% cross product
%
    
function c = cross(a,b)
    c = [a(2).*b(3)-a(3).*b(2), a(3).*b(1)-a(1).*b(3), a(1).*b(2)-a(2).*b(1)];
    
%
% Trigonometric functions for fi
%

function y = sin(x)
    if x < pi/2
        [y,t] = fi_sin_cos(x);
    else
        [y0,t] = fi_sin_cos(x-pi);
        y = -y0;
    end
        
function y = cos(x)
    if x < pi/2
        [t,y] = fi_sin_cos(x);
    else
        [t,y0] = fi_sin_cos(x-pi);
        y = -y0;
    end

function [scale,ks,phases] = cordic_table
    m = fimath('MaxProductWordLength',32,'MaxSumWordLength',32,...
                   'ProductFractionLength',28,'ProductMode','SpecifyPrecision',...
                   'SumFractionLength',28,'SumMode','SpecifyPrecision');
    t = numerictype(1,32,28);
    k0 = fi(2^0,t,m);
    p0 = atan(double(k0));
    k1 = fi(2^-1,t,m);
    p1 = atan(double(k1));
    k2 = fi(2^-2,t,m);
    p2 = atan(double(k2));
    k3 = fi(2^-3,t,m);
    p3 = atan(double(k3));
    k4 = fi(2^-4,t,m);
    p4 = atan(double(k4));
    k5 = fi(2^-5,t,m);
    p5 = atan(double(k5));
    k6 = fi(2^-6,t,m);
    p6 = atan(double(k6));
    k7 = fi(2^-7,t,m);
    p7 = atan(double(k7));
    k8 = fi(2^-8,t,m);
    p8 = atan(double(k8));
    k9 = fi(2^-9,t,m);
    p9 = atan(double(k9));
    k10 = fi(2^-10,t,m);
    p10 = atan(double(k10));
    k11 = fi(2^-11,t,m);
    p11 = atan(double(k11));
    k12 = fi(2^-12,t,m);
    p12 = atan(double(k12));
    k13 = fi(2^-13,t,m);
    p13 = atan(double(k13));
    k14 = fi(2^-14,t,m);
    p14 = atan(double(k14));
    ks = [k0 k1 k2 k3 k4 k5 k6 k7 k8 k9 k10 k11 k12 k13 k14];
    phases = fi([p0 p1 p2 p3 p4 p5 p6 p7 p8 p9 p10 p11 p12 p13 p14],t,m);

    p = fi(0,t,m);
    z = fi(complex(1,0),t,m);
    for i=1:length(ks)
        if imag(z) >= 0.0
            z = complex(real(z)+imag(z)*ks(i),...
                        imag(z)-real(z)*ks(i));
            p = p + phases(i);
        else
            z = complex(real(z)-imag(z)*ks(i),...
                        imag(z)+real(z)*ks(i));
            p = p - phases(i);
        end
    end
    scale = divide(t,1,real(z));
    
function [sin_x,cos_x] = fi_sin_cos(x)
    [scale,ks,phases] = cordic_table;
    t = numerictype(scale);
    m = fimath(scale);
    p = fi(0,t,m);
    if x > pi/2
        z = fi(complex(0,1),t,m);
        p = fi(pi/2,t,m);
    elseif x < -pi/2
        z = fi(complex(0,-1),t,m);
        p = fi(-pi/2,t,m);
    else
        z = fi(complex(1,0),t,m);
        p = fi(0,t,m);
    end
    for i = 1:length(ks)
        if x < p
            z = complex(real(z)+imag(z)*ks(i),...
                        imag(z)-real(z)*ks(i));
            p = p - phases(i);
        else
            z = complex(real(z)-imag(z)*ks(i),...
                        imag(z)+real(z)*ks(i));
            p = p + phases(i);
        end
    end
    sin_x = fi(imag(z) * scale,numerictype(x),fimath(x));
    cos_x = fi(real(z) * scale,numerictype(x),fimath(x));
